simulink model "l14_5"  (R2018b)
settings: Solver=ode45  StartTime=0  StopTime=200  MaxStep=5e-5  MinStep=1e-6  RelTol=1e-6  AbsTol=1e-4  EnableMultiTasking=on
settings Model: Creator=Joe  LastModifiedBy=joema
settings SolverCC: AutoScaleAbsTol=off
settings DataIOCC: LimitDataPoints=on  SaveFormat=Array
settings OptimizationCC: LifeSpan=inf
settings DebuggingCC: UnderspecifiedInitializationDetection=Classic  MergeDetectMultiDrivingBlocksExec=none  SolverPrmCheckMsg=warning  LibraryContextMissingDiagnostic=none  SFUnexpectedBacktrackingDiag=warning  SFNoUnconditionalDefaultTransitionDiag=warning  SFExecutionAtInitializationDiag=none
settings HardwareCC: ProdBitPerPointer=32  ProdBitPerSizeT=32  ProdBitPerPtrDiffT=32  ProdLargestAtomicFloat=None  ProdIntDivRoundTo=Undefined  ProdEndianess=Unspecified  ProdWordSize=32  ProdHWDeviceType=32-bit Generic
settings ModelReferenceCC: PropagateSignalLabelsOutOfModel=off
settings SFSimCC: SimUseLocalCustomCode=off
settings RTWCC: RTWUseLocalCustomCode=off
settings CodeAppCC: StateflowObjectComments=on
settings GRTTargetCC: TargetLangStandard=C89/C90 (ANSI)  GeneratePreprocessorConditionals=Disable all
settings ConfigComp: CovMetricSettings=dw  CovHtmlReporting=on  CovSaveCumulativeToWorkspaceVar=on  CovSaveSingleToWorkspaceVar=on  CovExternalEMLEnable=off  CovSFcnEnable=off

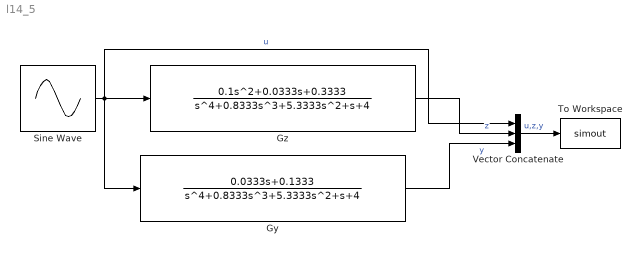
== system l14_5 ==
  Gy : TransferFcn  Numerator="[0.0333    0.1333]"  Denominator="[    1    0.8333    5.3333    1.    4]"
  Gz : TransferFcn  Numerator="[  0.1    0.0333    0.3333]"  Denominator="[    1    0.8333    5.3333    1.    4]"
  Sine Wave : Sin  Amplitude=2000  Frequency=5  SampleTime=0
  To Workspace : ToWorkspace  VariableName=simout  SaveFormat=Timeseries  SampleTime=-1
  Vector Concatenate : Concatenate  NumInputs=3
  wires:
  Sine Wave/1 -> Gy/1, Vector Concatenate/1, Gz/1  "u"
  Gy/1 -> Vector Concatenate/3  "y"
  Gz/1 -> Vector Concatenate/2  "z"
  Vector Concatenate/1 -> To Workspace/1  "u,z,y"
